simulink library "hyperbolic_saturation"  (R2022a)
settings: Solver=VariableStepAuto  StartTime=0.0  StopTime=10.0  RelTol=1e-3
settings Model: Creator=Niccolò  LastModifiedBy=Niccolò

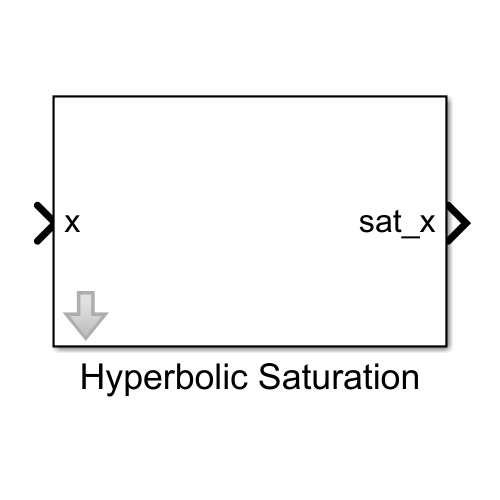
[thumbnail: Simulink's stored preview of the top-level diagram]
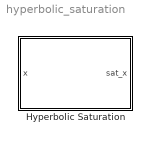
== system hyperbolic_saturation ==
  Hyperbolic Saturation : Subsystem  mask{amplitude=1, saturation=1}

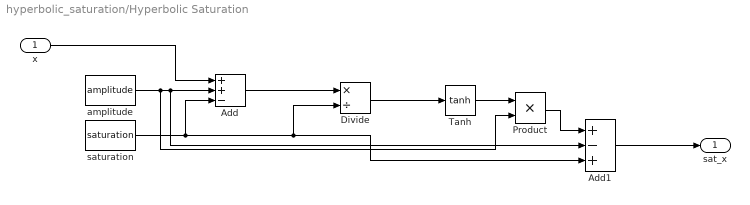
== system hyperbolic_saturation/Hyperbolic Saturation ==
  x : Inport
  Add : Sum  Inputs=++-
  Add1 : Sum  Inputs=+-+
  Divide : Product  Inputs=*/
  Product : Product
  Tanh : Trigonometry  Operator=tanh
  amplitude : Constant  Value=amplitude
  saturation : Constant  Value=saturation
  sat_x : Outport
  wires:
  saturation/1 -> Divide/2, Add1/3, Add/3
  Add/1 -> Divide/1
  amplitude/1 -> Add1/2, Add/2, Product/2
  Divide/1 -> Tanh/1
  Add1/1 -> sat_x/1
  Product/1 -> Add1/1
  Tanh/1 -> Product/1
  x/1 -> Add/1
